simulink model "basic_spring_mass_damper"  (R2019a)
settings: Solver=VariableStepAuto  StartTime=0.0  StopTime=100  RelTol=1e-3
undefined symbols (not defined in the file): A, b, epsilon, f_k, k, M, N
settings Model: Creator=Lenovo  LastModifiedBy=Lenovo
settings DataIOCC: ReturnWorkspaceOutputs=off
settings DebuggingCC: ArithmeticOperatorsInVariantConditions=warning

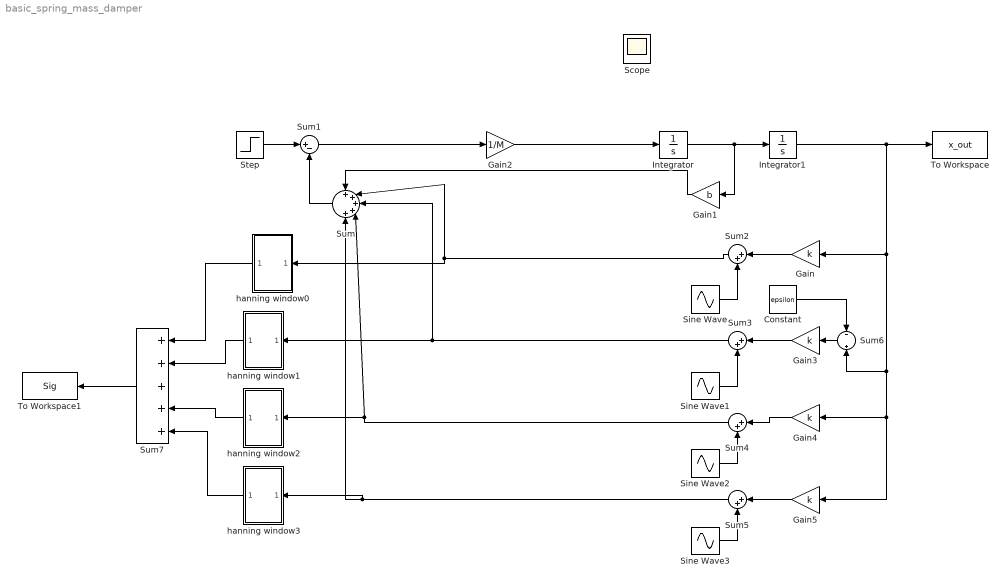
== system basic_spring_mass_damper ==
  Constant : Constant  Value=epsilon
  Gain{,3..5} (4 alike) : Gain  Gain=k
  Gain1 : Gain  Gain=b
  Gain2 : Gain  Gain=1/M
  Integrator : Integrator
  Integrator1 : Integrator
  Sine Wave{,1..3} (4 alike) : Sin  Amplitude=A  Frequency=pi*2*f_k  SampleTime=0.001
  Step : Step  After=0.01  SampleTime=0.001
  Sum : Sum  Inputs=+++++
  Sum1 : Sum  Inputs=|+-
  Sum{2..5} (4 alike) : Sum  Inputs=|++
  Sum6 : Sum  Inputs=-||+
  Sum7 : Sum  Inputs=+++++
  To Workspace : ToWorkspace  VariableName=x_out  SaveFormat=Timeseries  SampleTime=-1
  To Workspace1 : ToWorkspace  VariableName=Sig  SaveFormat=Timeseries  SampleTime=-1
  hanning window0 : Subsystem
  hanning window1 : Subsystem
  hanning window2 : Subsystem
  hanning window3 : Subsystem
  Scope : Scope
  wires:
  Integrator/1 -> Gain1/1, Integrator1/1
  Gain1/1 -> Sum/1
  Sum/1 -> Sum1/2
  Sum1/1 -> Gain2/1
  Step/1 -> Sum1/1
  Gain2/1 -> Integrator/1
  Gain/1 -> Sum2/1
  Sine Wave/1 -> Sum2/2
  Gain3/1 -> Sum3/1
  Sine Wave1/1 -> Sum3/2
  Gain4/1 -> Sum4/1
  Sine Wave2/1 -> Sum4/2
  Gain5/1 -> Sum5/1
  Integrator1/1 -> To Workspace/1, Sum6/2, Gain5/1, Gain4/1, Gain/1
  Sine Wave3/1 -> Sum5/2
  Sum6/1 -> Gain3/1
  Constant/1 -> Sum6/1
  Sum5/1 -> hanning window3/1(In1), Sum/5
  Sum4/1 -> Sum/4, hanning window2/1(In1)
  Sum3/1 -> hanning window1/1(In1), Sum/3
  Sum2/1 -> hanning window0/1(In1), Sum/2
  hanning window0/1(Out1) -> Sum7/1
  hanning window2/1(Out1) -> Sum7/4
  hanning window3/1(Out1) -> Sum7/5
  Sum7/1 -> To Workspace1/1
  hanning window1/1(Out1) -> Sum7/2

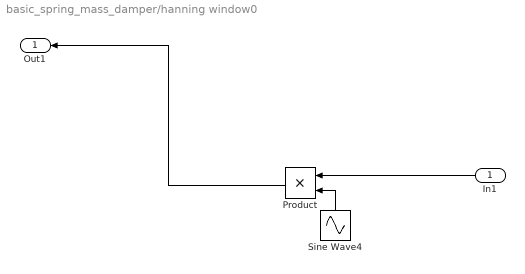
== system basic_spring_mass_damper/hanning window0 ==
  In1 : Inport
  Product : Product
  Sine Wave4 : Sin  Amplitude=0.5  Bias=0.5  Frequency=f_k*2*pi/N  Phase=pi*2/4*0  SampleTime=0
  Out1 : Outport
  wires:
  Product/1 -> Out1/1
  Sine Wave4/1 -> Product/2
  In1/1 -> Product/1

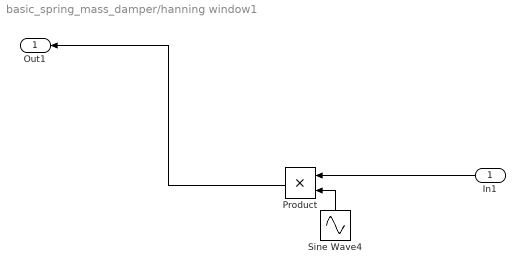
== system basic_spring_mass_damper/hanning window1 ==
  In1 : Inport
  Product : Product
  Sine Wave4 : Sin  Amplitude=0.5  Bias=0.5  Frequency=f_k*2*pi/N  Phase=pi*2/4*1  SampleTime=0
  Out1 : Outport
  wires:
  Product/1 -> Out1/1
  Sine Wave4/1 -> Product/2
  In1/1 -> Product/1

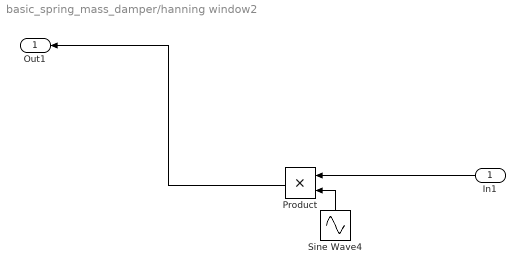
== system basic_spring_mass_damper/hanning window2 ==
  In1 : Inport
  Product : Product
  Sine Wave4 : Sin  Amplitude=0.5  Bias=0.5  Frequency=f_k*2*pi/N  Phase=pi*2/4*2  SampleTime=0
  Out1 : Outport
  wires:
  Product/1 -> Out1/1
  Sine Wave4/1 -> Product/2
  In1/1 -> Product/1

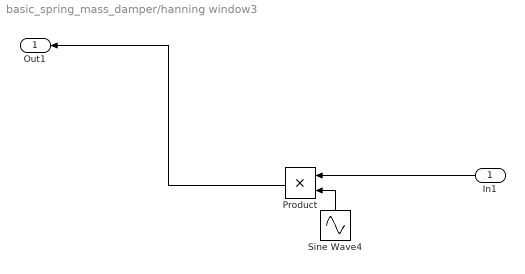
== system basic_spring_mass_damper/hanning window3 ==
  In1 : Inport
  Product : Product
  Sine Wave4 : Sin  Amplitude=0.5  Bias=0.5  Frequency=f_k*2*pi/N  Phase=pi*2/4*3  SampleTime=0
  Out1 : Outport
  wires:
  Product/1 -> Out1/1
  Sine Wave4/1 -> Product/2
  In1/1 -> Product/1
